simulink model "LCK_DanishV01"  (R2018b)
settings: Solver=FixedStepDiscrete  StartTime=0.0  StopTime=inf  FixedStep=0.01  RelTol=1e-3
PostLoadFcn:
  | if any(exist('dsrtsu_mdlpostloadfcn', 'file') ~= 0), dsrtsu_mdlpostloadfcn('Execute', bdroot); end
values from neighbouring files (symbols this model uses):
  C_DEG2RAD = 0.0175    [LCK_Macro.sldd]
  C_KPH2MPS = 0.2778    [LCK_Macro.sldd]
  C_NEARZERO = 0.0001    [LCK_Macro.sldd]
  C_ONE = 1.0    [LCK_Macro.sldd]
  C_RAD2DEG = 57.2958    [LCK_Macro.sldd]
  C_ZERO = 0.0    [LCK_Macro.sldd]
  k_accel_pedal_pos_per_speed_x : value not decoded    [LCK_LogicPara.sldd]
  k_accel_pedal_pos_per_speed_z : value not decoded    [LCK_LogicPara.sldd]
  k_brake_suprress_hold = 1000.0    [LCK_LogicPara.sldd]
  k_driver_appl_torque_filt = 50.0    [LCK_LogicPara.sldd]
  k_driver_suppression_hold_time = 3000.0    [LCK_LogicPara.sldd]
  k_hands_on_wheel_hold_msec = 500.0    [LCK_LogicPara.sldd]
  k_hands_on_wheel_torque_hi = 0.2    [LCK_LogicPara.sldd]
  k_hands_on_wheel_torque_lo = 0.15    [LCK_LogicPara.sldd]
  k_handsoff_delay_cycles = 50.0    [LCK_LogicPara.sldd]
  k_handsoff_torq_Lo_CR = 0.3    [LCK_LogicPara.sldd]
  k_handson_delay_cycles = 5.0    [LCK_LogicPara.sldd]
  k_HighAccel_suppress_hold = 3000.0    [LCK_LogicPara.sldd]
  k_HLR_suprress_hold = 3000.0    [LCK_LogicPara.sldd]
  k_hs_StrAng_CR_threshold_z : value not decoded    [LCK_LogicPara.sldd]
  k_LC_Exit_Switch = 0.0    [LCK_LogicPara.sldd]
  k_LCG_Configured = 1.0    [LCK_LogicPara.sldd]
  k_LCK_A0_Rdy2Act_UseConst = 0.0    [LCK_LogicPara.sldd]
  k_LCK_A0Fac_ActSta : value not decoded    [LCK_CtrlPara.sldd]
  k_LCK_A0Fac_DrvStm : value not decoded    [LCK_CtrlPara.sldd]
  k_LCK_A0Shift_LftCurv : value not decoded    [LCK_CtrlPara.sldd]
  k_LCK_A0Shift_RgtCurv : value not decoded    [LCK_CtrlPara.sldd]
  k_LCK_A0Shift_StraLan = 0.0    [LCK_CtrlPara.sldd]
  k_LCK_A0ShiftFac_Dy_LftCurv : value not decoded    [LCK_CtrlPara.sldd]
  k_LCK_A0ShiftFac_Dy_RgtCurv : value not decoded    [LCK_CtrlPara.sldd]
  k_LCK_A0ShiftFac_Vspd : value not decoded    [LCK_CtrlPara.sldd]
  k_LCK_accel_inhibit_thold = 35.0    [LCK_LogicPara.sldd]
  k_LCK_Active2Ready_Mask = 255.0    [LCK_LogicPara.sldd]
  k_LCK_CvatRateBks : value not decoded    [LCK_CtrlPara.sldd]
  k_LCK_CvatrBks : value not decoded    [LCK_CtrlPara.sldd]
  k_LCK_DFac_Dy : value not decoded    [LCK_CtrlPara.sldd]
  k_LCK_DFac_Dy_Curv : value not decoded    [LCK_CtrlPara.sldd]
  k_LCK_DFac_HaCurCen : value not decoded    [LCK_CtrlPara.sldd]
  k_LCK_DFac_HaCurSid : value not decoded    [LCK_CtrlPara.sldd]
  k_LCK_DFac_HadCurCen : value not decoded    [LCK_CtrlPara.sldd]
  k_LCK_DFac_HadCurSid : value not decoded    [LCK_CtrlPara.sldd]
  k_LCK_DFac_HadStrCen : value not decoded    [LCK_CtrlPara.sldd]
  k_LCK_DFac_HadStrSid : value not decoded    [LCK_CtrlPara.sldd]
  k_LCK_DFac_HaStrCen : value not decoded    [LCK_CtrlPara.sldd]
  k_LCK_DFac_HaStrSid : value not decoded    [LCK_CtrlPara.sldd]
  k_LCK_DFac_Rad : value not decoded    [LCK_CtrlPara.sldd]
  k_LCK_DFac_SA_CurCen : value not decoded    [LCK_CtrlPara.sldd]
  k_LCK_DFac_SA_CurSid : value not decoded    [LCK_CtrlPara.sldd]
  k_LCK_DFac_SA_StrCen : value not decoded    [LCK_CtrlPara.sldd]
  k_LCK_DFac_SA_StrSid : value not decoded    [LCK_CtrlPara.sldd]
  k_LCK_DFac_SS_CurCen : value not decoded    [LCK_CtrlPara.sldd]
  k_LCK_DFac_SS_CurSid : value not decoded    [LCK_CtrlPara.sldd]
  k_LCK_DFac_SS_StrCen : value not decoded    [LCK_CtrlPara.sldd]
  k_LCK_DFac_SS_StrSid : value not decoded    [LCK_CtrlPara.sldd]
  k_LCK_DFac_Vspd : value not decoded    [LCK_CtrlPara.sldd]
  k_LCK_DlyTm_DrvStim = 0.2    [LCK_CtrlPara.sldd]
  k_LCK_DTermMax = 2.0    [LCK_CtrlPara.sldd]
  k_LCK_DyBks_Curv : value not decoded    [LCK_CtrlPara.sldd]
  k_LCK_Enable_POOnly = 1.0    [LCK_LogicPara.sldd]
  k_LCK_Entry_DistBuffer = 0.1    [LCK_LogicPara.sldd]
  k_LCK_Fac_Vspd2RngThr_FalRec = 0.23    [LCK_CtrlPara.sldd]
  k_LCK_Ffw_CvatSwh = 0.0    [LCK_CtrlPara.sldd]
  k_LCK_Ffw_DyBks : value not decoded    [LCK_CtrlPara.sldd]
  k_LCK_Ffw_TimCon_CmdFlt = 0.0    [LCK_CtrlPara.sldd]
  k_LCK_FfwDeltaFac_Rad_Lft : value not decoded    [LCK_CtrlPara.sldd]
  k_LCK_FfwDeltaFac_Rad_Rgt : value not decoded    [LCK_CtrlPara.sldd]
  k_LCK_FfwDeltaFac_Vspd : value not decoded    [LCK_CtrlPara.sldd]
  k_LCK_FfwFac_CvatRate_Lft : value not decoded    [LCK_CtrlPara.sldd]
  k_LCK_FfwFac_CvatRate_Rgt : value not decoded    [LCK_CtrlPara.sldd]
  k_LCK_FfwFac_Dy : value not decoded    [LCK_CtrlPara.sldd]
  k_LCK_FfwFac_Rad_Lft : value not decoded    [LCK_CtrlPara.sldd]
  k_LCK_FfwFac_Rad_Rgt : value not decoded    [LCK_CtrlPara.sldd]
  k_LCK_FfwFac_Vspd : value not decoded    [LCK_CtrlPara.sldd]
  k_LCK_FfwTorq_Cvat : value not decoded    [LCK_CtrlPara.sldd]
  k_LCK_HAFac_ActSta : value not decoded    [LCK_CtrlPara.sldd]
  k_LCK_HAFac_DrvStm : value not decoded    [LCK_CtrlPara.sldd]
  k_LCK_HaloTime = 2000.0    [LCK_LogicPara.sldd]
  k_LCK_HaloTime_Switch = 0.0    [LCK_LogicPara.sldd]
  k_LCK_HARFac_ActSta : value not decoded    [LCK_CtrlPara.sldd]
  k_LCK_HARFac_DrvStm : value not decoded    [LCK_CtrlPara.sldd]
  k_LCK_Hed_DyBks : value not decoded    [LCK_CtrlPara.sldd]
  k_LCK_HedAngDiffX : value not decoded    [LCK_CtrlPara.sldd]
  k_LCK_HedAngRateDiffX : value not decoded    [LCK_CtrlPara.sldd]
  k_LCK_HndsOnWhel_DlyTm_Idl2Rdy = 0.0    [LCK_LogicPara.sldd]
  k_LCK_host_veh_width = 1.86    [LCK_LogicPara.sldd]
  k_LCK_Idle2Ready_Mask = 239.0    [LCK_LogicPara.sldd]
  k_LCK_Junc_SusTime = 1.0    [LCK_LogicPara.sldd]
  k_LCK_KpKdDecSlopeLmt = 10.0    [LCK_CtrlPara.sldd]
  k_LCK_KpKdIncSlopeLmt = 5.0    [LCK_CtrlPara.sldd]
  k_LCK_Lat_Ctrl_DFac_Lft = 1.0    [LCK_CtrlPara.sldd]
  k_LCK_Lat_Ctrl_DFac_Rgt = 1.05    [LCK_CtrlPara.sldd]
  k_LCK_Lat_Ctrl_Kd = 0.8    [LCK_CtrlPara.sldd]
  k_LCK_Lat_Ctrl_Ki = 0.5    [LCK_CtrlPara.sldd]
  k_LCK_Lat_Ctrl_Kp = 0.7    [LCK_CtrlPara.sldd]
  k_LCK_Lat_Ctrl_Kp_NearGain = 0.7    [LCK_CtrlPara.sldd]
  k_LCK_Lat_Ctrl_PFac_Lft = 1.0    [LCK_CtrlPara.sldd]
  k_LCK_Lat_Ctrl_PFac_Rgt = 1.05    [LCK_CtrlPara.sldd]
  k_LCK_Lat_Ctrl_TimCon_CmdFlt = 5.0    [LCK_CtrlPara.sldd]
  k_LCK_Lat_DFac_Rad : value not decoded    [LCK_CtrlPara.sldd]
  k_LCK_Lat_DFac_SS_Cur : value not decoded    [LCK_CtrlPara.sldd]
  k_LCK_Lat_DFac_SS_Str : value not decoded    [LCK_CtrlPara.sldd]
  k_LCK_Lat_DFac_Vspd : value not decoded    [LCK_CtrlPara.sldd]
  k_LCK_Lat_DyBks : value not decoded    [LCK_CtrlPara.sldd]
  k_LCK_Lat_IFac_Rad : value not decoded    [LCK_CtrlPara.sldd]
  k_LCK_Lat_IFac_Vspd : value not decoded    [LCK_CtrlPara.sldd]
  k_LCK_Lat_ILmtFac_Dy_CurvLan : value not decoded    [LCK_CtrlPara.sldd]
  k_LCK_Lat_ILmtFac_Dy_StraLan : value not decoded    [LCK_CtrlPara.sldd]
  k_LCK_Lat_ILmtFac_Rad : value not decoded    [LCK_CtrlPara.sldd]
  k_LCK_Lat_ILmtFac_Rad_NearGain = 1.0    [LCK_CtrlPara.sldd]
  k_LCK_Lat_ILmtFac_Vspd_CurvLan : value not decoded    [LCK_CtrlPara.sldd]
  k_LCK_Lat_ILmtFac_Vspd_StraLan : value not decoded    [LCK_CtrlPara.sldd]
  k_LCK_Lat_ITermLmt_Dy = 1.0    [LCK_CtrlPara.sldd]
  k_LCK_Lat_KpKdDecSlopeLmt = 10.0    [LCK_CtrlPara.sldd]
  k_LCK_Lat_KpKdIncSlopeLmt = 10.0    [LCK_CtrlPara.sldd]
  k_LCK_Lat_PFac_Dy_InnLftCur : value not decoded    [LCK_CtrlPara.sldd]
  k_LCK_Lat_PFac_Dy_InnRgtCur : value not decoded    [LCK_CtrlPara.sldd]
  k_LCK_Lat_PFac_Dy_OutLftCur : value not decoded    [LCK_CtrlPara.sldd]
  k_LCK_Lat_PFac_Dy_OutRgtCur : value not decoded    [LCK_CtrlPara.sldd]
  k_LCK_Lat_PFac_Dy_Str : value not decoded    [LCK_CtrlPara.sldd]
  k_LCK_Lat_PFac_Rad : value not decoded    [LCK_CtrlPara.sldd]
  ... (+153 more)
undefined symbols (not defined in the file or in its folder): k_LCK_CurvBks, K_LCK_SPA0A1A2_LMRngCmp_y
libraries: LateralControl_fcns_lib x58, simulink x24
(part 14 of 47)

== system LCK_DanishV01/Lateral_Control_Module/Steer_Path_Process/Calculation_of_SPP_Confidence ==
  Lin01_Prob_Fltd : Inport
  Lin02_Prob_Fltd : Inport  Port=2
  Constant : Constant  Value=k_LCK_SPPConfHigh_ProbThre
  Constant1 : Constant  Value=4
  Constant2 : Constant  Value=k_LCK_SPPConfMedHigh_ProbThre
  Constant3 : Constant  Value=3
  Constant4 : Constant  Value=k_LCK_SPPConfMed_ProbThre
  Constant5 : Constant  Value=2
  Constant6 : Constant
  Constant7 : Constant  Value=k_LCK_SPPConfHigh_ProbThre
  Constant8 : Constant  Value=k_LCK_SPPConfMedHigh_ProbThre
  Constant9 : Constant  Value=k_LCK_SPPConfMed_ProbThre
  Logical Operator : Logic  AllPortsSameDT=off  OutDataTypeStr=boolean
  Logical Operator1 : Logic  AllPortsSameDT=off  OutDataTypeStr=boolean
  Logical Operator2 : Logic  AllPortsSameDT=off  OutDataTypeStr=boolean
  Relational Operator{,1..5} (6 alike) : RelationalOperator  OutDataTypeStr=boolean  RndMeth=Simplest
  Switch : Switch  Criteria=u2 > Threshold
  Switch1 : Switch  Criteria=u2 > Threshold
  Switch2 : Switch  Criteria=u2 > Threshold
  SPP_Conf_Raw : Outport
  wires:
  Constant6/1 -> Switch2/3
  Lin01_Prob_Fltd/1 -> Relational Operator/1, Relational Operator2/1, Relational Operator1/1
  Logical Operator1/1 -> Switch1/2
  Logical Operator2/1 -> Switch2/2
  Constant8/1 -> Relational Operator4/2
  Constant/1 -> Relational Operator/2
  Logical Operator/1 -> Switch/2
  Constant9/1 -> Relational Operator5/2
  Relational Operator5/1 -> Logical Operator2/2
  Constant3/1 -> Switch1/1
  Constant2/1 -> Relational Operator1/2
  Constant1/1 -> Switch/1
  Relational Operator2/1 -> Logical Operator2/1
  Constant4/1 -> Relational Operator2/2
  Lin02_Prob_Fltd/1 -> Relational Operator3/1, Relational Operator5/1, Relational Operator4/1
  Constant7/1 -> Relational Operator3/2
  Constant5/1 -> Switch2/1
  Relational Operator/1 -> Logical Operator/1
  Relational Operator1/1 -> Logical Operator1/1
  Relational Operator3/1 -> Logical Operator/2
  Switch2/1 -> Switch1/3
  Switch1/1 -> Switch/3
  Relational Operator4/1 -> Logical Operator1/2
  Switch/1 -> SPP_Conf_Raw/1

== system LCK_DanishV01/Lateral_Control_Module/Steer_Path_Process/Calculation_of_SPP_Type ==
  Lin01_Type : Inport
  Lin02_Type : Inport  Port=2
  Constant{10..14,18..19,23..24,28} (10 alike) : Constant  Value=0
  Constant{15..16,20..21,25..26} (6 alike) : Constant  Value=4
  Constant17 : Constant
  Constant22 : Constant  Value=2
  Constant27 : Constant  Value=3
  Logical Operator{3..4,6..7,9..12} (8 alike) : Logic  AllPortsSameDT=off  OutDataTypeStr=boolean
  Logical Operator5 : Logic  Operator=OR  AllPortsSameDT=off  OutDataTypeStr=boolean
  Logical Operator8 : Logic  Operator=OR  AllPortsSameDT=off  OutDataTypeStr=boolean
  Relational Operator{8,10,12,14,16..19} (8 alike) : RelationalOperator  Operator=>  OutDataTypeStr=boolean  RndMeth=Simplest
  Relational Operator{6..7,11,13} (4 alike) : RelationalOperator  Operator===  OutDataTypeStr=boolean  RndMeth=Simplest
  Relational Operator15 : RelationalOperator  Operator=<=  OutDataTypeStr=boolean  RndMeth=Simplest
  Relational Operator9 : RelationalOperator  Operator=<=  OutDataTypeStr=boolean  RndMeth=Simplest
  Switch{3..6} (4 alike) : Switch  Criteria=u2 > Threshold
  SPP_Type_Raw : Outport
  wires:
  Logical Operator9/1 -> Switch5/2
  Constant12/1 -> Switch3/1
  Constant15/1 -> Relational Operator10/1
  Constant11/1 -> Relational Operator7/2
  Constant26/1 -> Relational Operator19/1
  Lin02_Type/1 -> Relational Operator7/1, Relational Operator9/2, Relational Operator11/1, Relational Operator12/2, Relational Operator14/1, Relational Operator19/2, Relational Operator17/1
  Logical Operator12/1 -> Switch6/2
  Relational Operator7/1 -> Logical Operator3/2
  Lin01_Type/1 -> Relational Operator6/1, Relational Operator13/1, Relational Operator15/2, Relational Operator16/2, Relational Operator18/1, Relational Operator10/2, Relational Operator8/1
  Relational Operator8/1 -> Logical Operator4/2
  Relational Operator14/1 -> Logical Operator7/2
  Relational Operator17/1 -> Logical Operator11/2
  Constant23/1 -> Relational Operator18/2
  Constant14/1 -> Relational Operator11/2
  Constant16/1 -> Relational Operator9/1
  Logical Operator11/1 -> Logical Operator12/2
  Constant21/1 -> Relational Operator15/1
  Logical Operator7/1 -> Logical Operator9/1
  Constant13/1 -> Relational Operator8/2
  Relational Operator11/1 -> Logical Operator5/2
  Logical Operator6/1 -> Switch4/2
  Logical Operator5/1 -> Logical Operator6/2
  Relational Operator6/1 -> Logical Operator3/1
  Constant19/1 -> Relational Operator13/2
  Relational Operator9/1 -> Logical Operator5/1
  Constant17/1 -> Switch4/1
  Switch5/1 -> Switch4/3
  Constant22/1 -> Switch5/1
  Relational Operator15/1 -> Logical Operator8/1
  Relational Operator16/1 -> Logical Operator10/1
  Switch4/1 -> Switch3/3
  Constant20/1 -> Relational Operator12/1
  Switch6/1 -> Switch5/3
  Constant25/1 -> Relational Operator16/1
  Constant24/1 -> Relational Operator17/2
  Logical Operator10/1 -> Logical Operator12/1
  Relational Operator19/1 -> Logical Operator11/1
  Constant27/1 -> Switch6/1
  Relational Operator10/1 -> Logical Operator4/1
  Relational Operator13/1 -> Logical Operator8/2
  Logical Operator8/1 -> Logical Operator9/2
  Relational Operator18/1 -> Logical Operator10/2
  Relational Operator12/1 -> Logical Operator7/1
  Constant18/1 -> Relational Operator14/2
  Logical Operator4/1 -> Logical Operator6/1
  Logical Operator3/1 -> Switch3/2
  Constant28/1 -> Switch6/3
  Constant10/1 -> Relational Operator6/2
  Switch3/1 -> SPP_Type_Raw/1

== system LCK_DanishV01/Lateral_Control_Module/Steer_Path_Process/Determination_of_SPP_Conf_and_Type ==
  Lin01_Invalid : Inport
  Lin02_Invalid : Inport  Port=2
  SPP_Conf_Raw : Inport  Port=3
  SPP_Type_Raw : Inport  Port=4
  Constant59 : Constant  Value=3
  Constant60 : Constant  Value=3
  Data Type Conversion : DataTypeConversion  OutDataTypeStr=single
  Data Type Conversion1 : DataTypeConversion  OutDataTypeStr=single
  Logical Operator25 : Logic  Operator=OR  AllPortsSameDT=off  OutDataTypeStr=boolean
  Switch7 : Switch  Criteria=u2 > Threshold
  Switch8 : Switch  Criteria=u2 > Threshold
  SPP_Conf : Outport
  SPP_Type : Outport  Port=2
  wires:
  Switch7/1 -> Data Type Conversion/1
  Logical Operator25/1 -> Switch7/2, Switch8/2
  SPP_Conf_Raw/1 -> Switch7/3
  Data Type Conversion1/1 -> SPP_Type/1
  SPP_Type_Raw/1 -> Switch8/3
  Switch8/1 -> Data Type Conversion1/1
  Constant60/1 -> Switch8/1
  Data Type Conversion/1 -> SPP_Conf/1
  Constant59/1 -> Switch7/1
  Lin02_Invalid/1 -> Logical Operator25/2
  Lin01_Invalid/1 -> Logical Operator25/1
